simulink model "controller_frf"  (R2017a)
settings: Solver=FixedStepAuto  StartTime=0.0  StopTime=SimTime  FixedStep=SampleTime  RelTol=1e-3
settings Model: Creator=marce  LastModifiedBy=marce

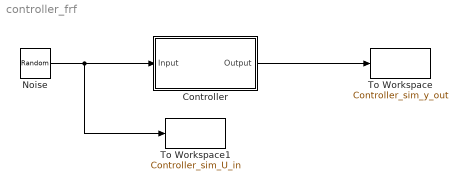
== system controller_frf ==
  Controller : Subsystem  mask(Controller){Kp=0.5, Kv=0.005, notch_zeros=59, notch_damping_zeros=0.03, notch_poles=59, notch_damping_poles=0.5, roll_off_poles=200, roll_off_damping_poles=0.5}
      mask prompts: notch_zeros "Notch zeros [Hz]"; notch_damping_zeros "Notch damping zeros [-]"; notch_poles "Notch poles [Hz]"; notch_damping_poles "Notch damping poles [-]"; roll_off_poles "Roll-off poles [Hz]"; roll_off_damping_poles "Roll-off damping poles [-]"
      mask help:
      | The controller consists of three filters: a Kp/Kv, a notch and a roll-off filter.
      | You can edit the parameters below.
  Noise : RandomNumber  Variance=0.1  SampleTime=0
  To Workspace : ToWorkspace  VariableName=Controller_sim_y_out  SaveFormat=Timeseries  SampleTime=-1
  To Workspace1 : ToWorkspace  VariableName=Controller_sim_U_in  SaveFormat=Timeseries  SampleTime=-1
  wires:
  Noise/1 -> To Workspace1/1, Controller/1(Input)
  Controller/1(Output) -> To Workspace/1

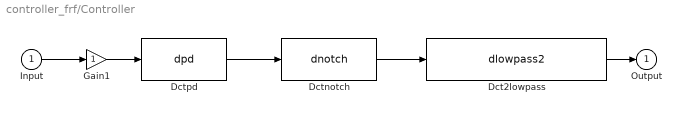
== system controller_frf/Controller ==
  Input : Inport
  Dct2lowpass : S-Function  FunctionName=dlowpass2  Parameters=f_den b_den 0.001  SFunctionDeploymentMode=off  EnableBusSupport=off  mask(dctools){f_den=roll_off_poles, b_den=roll_off_damping_poles}
      mask prompts: f_den "Pole [Hz]"; b_den "Damping pole [-]"
      mask help: This block implements a discrete time 2nd order lowpass filter.
      mask Display: disp('DCT 2nd order lowpass')
  Dctnotch : S-Function  FunctionName=dnotch  Parameters=f_num b_num f_den b_den 0.001  SFunctionDeploymentMode=off  EnableBusSupport=off  mask(dctools){f_num=notch_zeros, b_num=notch_damping_zeros, f_den=notch_poles, b_den=notch_damping_poles}
      mask prompts: f_num "Zero [Hz]"; b_num "Damping zero [-]"; f_den "Pole [Hz]"; b_den "Damping pole [-]"
      mask help: This block implements a dicrete time 2nd order notch filter.
      mask Display: disp('DCT notch')
  Dctpd : S-Function  FunctionName=dpd  Parameters=kp kv 0.001  SFunctionDeploymentMode=off  EnableBusSupport=off  mask(dctools){kp=Kp, kv=Kv}
      mask help: This block implements a discrete time pd filter.
      mask Display: disp('DCT pd')
  Gain1 : Gain  SaturateOnIntegerOverflow=on  OutDataTypeStr=Inherit: Same as input  ParamDataTypeStr=Inherit: Same as input
  Output : Outport
  wires:
  Dct2lowpass/1 -> Output/1
  Gain1/1 -> Dctpd/1
  Input/1 -> Gain1/1
  Dctpd/1 -> Dctnotch/1
  Dctnotch/1 -> Dct2lowpass/1
